simulink model "v7"  (R2023a)
settings: Solver=FixedStepAuto  StartTime=0.0  StopTime=Inf  RelTol=1e-3  EnableMultiTasking=on
undefined symbols (not defined in the file or in its folder): InputPWM, WheelSpeed
libraries: arduinolib x11, simulink x8, slpidlib x1, mobileRoboticsTrainingLib x1, arduinosensorlib x1
settings Model: ExtModeTrigDuration=2  Creator=friso  LastModifiedBy=friso
settings OptimizationCC: EnhancedBackFolding=on  PassReuseOutputArgsAs=Individual arguments  ZeroExternalMemoryAtStartup=off  ZeroInternalMemoryAtStartup=off  MaxStackSize=64  OptimizeBlockOrder=speed  DifferentSizesBufferReuse=on  OptimizationCustomize=off  EfficientTunableParamExpr=on
settings DebuggingCC: ParameterTunabilityLossMsg=error  UnderSpecifiedDimensionMsg=warning
settings HardwareCC: ProdBitPerPointer=32  ProdBitPerSizeT=32  ProdBitPerPtrDiffT=32  ProdLargestAtomicInteger=Long  ProdLargestAtomicFloat=Double  ProdWordSize=32  ProdHWDeviceType=ARM Compatible->ARM Cortex  UseEmbeddedCoderFeatures=off
settings SFSimCC: MATLABDynamicMemAlloc=off
settings RTWCC: Description=Embedded Coder  SystemTargetFile=ert.tlc  HardwareBoard=Arduino Nano 33 IoT  TemplateMakefile=ert_default_tmf  Toolchain=Arduino ARM  BuildConfiguration=Faster Runs
settings CodeAppCC: ForceParamTrailComments=on  IgnoreCustomStorageClasses=off  OperatorAnnotations=on  SimulinkDataObjDesc=on  SFDataObjDesc=on  InsertBlockDesc=on
settings ERTTargetCC: SupportContinuousTime=on  SupportNonInlinedSFcns=on  SupportVariableSizeSignals=on  ExtModeTransport=3  ExtModeStaticAlloc=on  ExtModeAutomaticAllocSize=off  ExtModeStaticAllocSize=8192  ExtModeMexFile=ext_xcp  ExtModeIntrfLevel=Level2 - Open

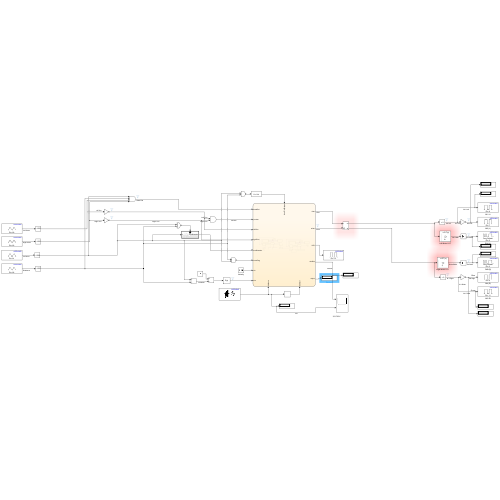
[thumbnail: Simulink's stored preview of the top-level diagram]
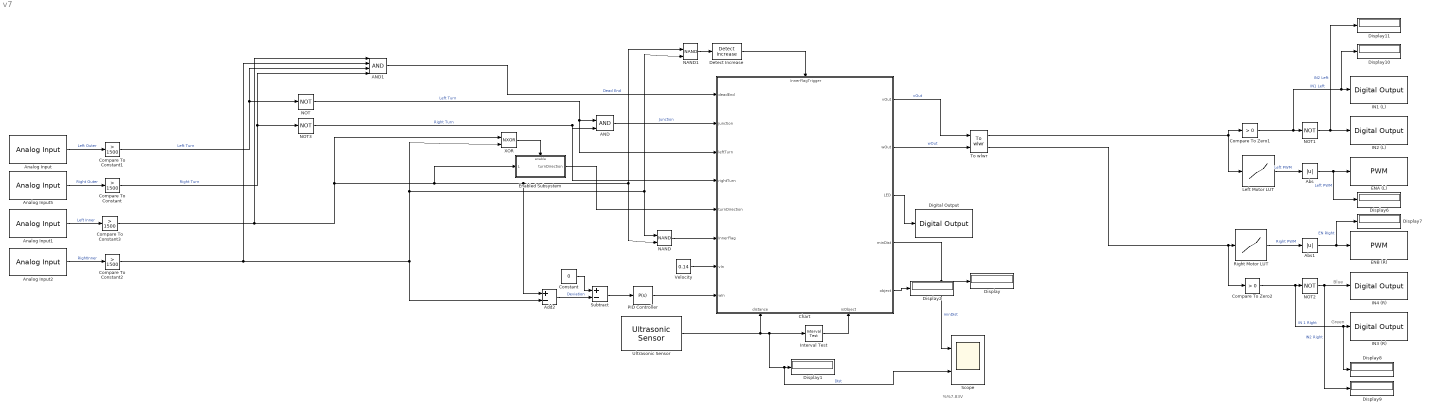
== system v7 ==
  note: %%7.83V
  note: Blue
  note: Green
  AND : Logic  IconShape=distinctive  AllPortsSameDT=off  OutDataTypeStr=boolean
  AND1 : Logic  Inputs=4  IconShape=distinctive  AllPortsSameDT=off  OutDataTypeStr=boolean
  Abs : Abs  SaturateOnIntegerOverflow=off
  Abs1 : Abs  SaturateOnIntegerOverflow=off
  Add2 : Sum  Inputs=+-  OutDataTypeStr=single
  Analog Input : arduinolib/Analog Input  pinNumber=0  ReadResultsOnly=off  ConversionTriggerSource=Software  ExternalTriggerType=uint32( 0 )  OutputDataType=uint16  EnableConversionCompleteNotify=off  EnableOuputStatus=off  SampleTime=-1  blockPlatform=arduino
  Analog Input1 : arduinolib/Analog Input  pinNumber=1  ReadResultsOnly=off  ConversionTriggerSource=Software  ExternalTriggerType=uint32( 0 )  OutputDataType=uint16  EnableConversionCompleteNotify=off  EnableOuputStatus=off  SampleTime=-1  blockPlatform=arduino
  Analog Input2 : arduinolib/Analog Input  pinNumber=2  ReadResultsOnly=off  ConversionTriggerSource=Software  ExternalTriggerType=uint32( 0 )  OutputDataType=uint16  EnableConversionCompleteNotify=off  EnableOuputStatus=off  SampleTime=-1  blockPlatform=arduino
  Analog Input5 : arduinolib/Analog Input  pinNumber=3  ReadResultsOnly=off  ConversionTriggerSource=Software  ExternalTriggerType=uint32( 0 )  OutputDataType=uint16  EnableConversionCompleteNotify=off  EnableOuputStatus=off  SampleTime=-1  blockPlatform=arduino
  Chart : Stateflow chart  TreatAsAtomicUnit=on
      settings: PortSchema="{\"entries\":[{\"content\":{\"sides\":[{\"content\":{\"connectorIds\":[\"In2\",\"In3\",\"In4\",\"In5\",\"In6\",\"In7\",\"In8\",\"In9\"]},\"type\":\"ConnectorPlacement.EquallySpacedRectSide\",\"uuid\":\"48d79888-744e-426e-80fd-4006989ca9f3\"},{\"content\":{\"connectorIds\":[\"Out2\",\"Out1\",\"Out3\",\"Out4\",\"Out5\"],\"side\":\"RIGHT\"},\"type\":\"ConnectorPlacement.EquallySpacedRectSide\",\"uuid\":\"a2b0e608-2864-4100-97ad-f114c331665e\"},{\"content\":{\"connectorIds\":[\"In1\"],\"side\":\"TOP\"},\"type\":\"ConnectorPlacement.EquallySpacedRectSide\",\"uuid\":\"9d579ed5-8468-4bce-b242-faef1fc44e90\"},{\"content\":{\"connectorIds\":[\"In11\",\"In10\"],\"side\":\"BOTTOM\"},\"type\":\"ConnectorPlacement.EquallySpacedRectSide\",\"uuid\":\"6fbdcd2a-7733-4dd1-bf5b-236cc3dcd5fd\"}]},\"type\":\"ConnectorPlacement.EquallySpacedConnector\",\"uuid\":\"bb2fff07-f9d5-40d5-a86f-bb5d79581747\"}],\"packageUris\":[\"http://schema.mathworks.com/mf0/Connector/R2020b\"],\"version\":\"1.0\"}"
  Compare To Constant{,1..3} (4 alike) : simulink/Logic and Bit Operations/Compare To Constant  relop=>  const=1500  OutDataTypeStr=uint8
  Compare To Zero1 : simulink/Logic and Bit Operations/Compare To Zero  relop=>  OutDataTypeStr=boolean
  Compare To Zero2 : simulink/Logic and Bit Operations/Compare To Zero  relop=>  OutDataTypeStr=boolean
  Constant : Constant  Value=0
  Detect Increase : simulink/Logic and Bit Operations/Detect Increase  vinit=0.0  OutDataTypeStr=boolean
  Digital Output : arduinolib/Digital Output  pinNumber=13  Direction=output  blockPlatform=arduino
  Display{,1..2,6..11} (9 alike) : Display
  ENA (L) : arduinolib/PWM  pinNumber=5  frequencyType=Default  desiredFrequency=490.2  achievableFrequency=490.2
  ENB (R) : arduinolib/PWM  pinNumber=3  frequencyType=Default  desiredFrequency=490.2  achievableFrequency=490.2
  Enabled Subsystem : Subsystem  TreatAsAtomicUnit=on
  IN1 (L) : arduinolib/Digital Output  pinNumber=9  Direction=output  blockPlatform=arduino
  IN2 (L) : arduinolib/Digital Output  pinNumber=7  Direction=output  blockPlatform=arduino
  IN3 (R) : arduinolib/Digital Output  pinNumber=11  Direction=output  blockPlatform=arduino
  IN4 (R) : arduinolib/Digital Output  pinNumber=6  Direction=output  blockPlatform=arduino
  Interval Test : simulink/Logic and Bit Operations/Interval Test  IntervalClosedRight=on  uplimit=0.5  IntervalClosedLeft=off  lowlimit=0  OutDataTypeStr=boolean
  Left Motor LUT : Lookup_n-D  NumberOfTableDimensions=1  BreakpointsForDimension1=WheelSpeed  Table=InputPWM  InterpMethod=Nearest  ExtrapMethod=Clip  InternalRulePriority=Speed  RndMeth=Simplest
  NAND : Logic  Operator=NAND  IconShape=distinctive  AllPortsSameDT=off  OutDataTypeStr=boolean
  NAND1 : Logic  Operator=NAND  IconShape=distinctive  AllPortsSameDT=off  OutDataTypeStr=boolean
  NOT{,1..3} (4 alike) : Logic  Operator=NOT  IconShape=distinctive  AllPortsSameDT=off  OutDataTypeStr=boolean
  PID Controller : slpidlib/PID Controller  Controller=P  Form=Parallel  TimeDomain=Continuous-time  UseExternalTs=off  SampleTime=-1  IntegratorMethod=Forward Euler  FilterMethod=Forward Euler  ControllerParametersSource=internal  P=0.87  I=1  UseKiTs=off  D=0  N=100  UseFilter=on  TunerSelectOption=Transfer Function Based (PID Tuner App)  InitialConditionSource=internal  InitialConditionForIntegrator=0  InitialConditionForFilter=0  DifferentiatorICPrevScaledInput=0  ExternalReset=none  TrackingMode=off  Kt=1  LimitOutput=off  SatLimitsSource=internal  UpperSaturationLimit=inf  LowerSaturationLimit=-inf  LinearizeAsGain=on  AntiWindupMode=none  Kb=1  LimitIntegrator=off  UpperIntegratorSaturationLimit=inf  LowerIntegratorSaturationLimit=-inf  POutMin=[]  POutMax=[]  IOutMin=[]  IOutMax=[]  DOutMin=[]  DOutMax=[]  NOutMin=[]  NOutMax=[]  SumOutMin=[]  SumOutMax=[]  SaturationOutMin=[]  SaturationOutMax=[]  PParamMin=[]  PParamMax=[]  IParamMin=[]  IParamMax=[]  DParamMin=[]  DParamMax=[]  NParamMin=[]  NParamMax=[]  KbParamMin=[]  KbParamMax=[]  KtParamMin=[]  KtParamMax=[]  KbOutMin=[]  KbOutMax=[]  KtOutMin=[]  KtOutMax=[]  IntegratorOutMin=[]  IntegratorOutMax=[]  FilterOutMin=[]  FilterOutMax=[]  SumI1OutMin=[]  SumI1OutMax=[]  SumI2OutMin=[]  SumI2OutMax=[]  SumI3OutMin=[]  SumI3OutMax=[]  SumI4OutMin=[]  SumI4OutMax=[]  SumDOutMin=[]  SumDOutMax=[]  DifferentiatorOutMin=[]  DifferentiatorOutMax=[]  FilterDiffOutCoefMin=[]  FilterDiffOutCoefMax=[]  ReciprocalOutMin=[]  ReciprocalOutMax=[]  SumDenOutMin=[]  SumDenOutMax=[]  SumNumOutMin=[]  SumNumOutMax=[]  DivideOutMin=[]  DivideOutMax=[]  UdiffTsProdOutMin=[]  UdiffTsProdOutMax=[]  NTsProdOutMin=[]  NTsProdOutMax=[]  UintegralTsProdOutMin=[]  UintegralTsProdOutMax=[]  UngainTsProdOutMin=[]  UngainTsProdOutMax=[]  ClampingZeroOutDataTypeStr=Inherit: Inherit via back propagation  ClampingZeroOutMin=[]  ClampingZeroOutMax=[]  FilterDenConstantOutDataTypeStr=Inherit: Inherit via back propagation  FilterDenConstantOutMin=[]  FilterDenConstantOutMax=[]  PCopyOutDataTypeStr=Inherit: Inherit via back propagation  PCopyOutMin=[]  PCopyOutMax=[]  NCopyOutDataTypeStr=Inherit: Inherit via back propagation  NCopyOutMin=[]  NCopyOutMax=[]  IntegratorContinuousStateAttributes=''  IntegratorStateMustResolveToSignalObject=off  IntegratorRTWStateStorageClass=Auto  FilterContinuousStateAttributes=''  FilterStateMustResolveToSignalObject=off  FilterRTWStateStorageClass=Auto  ParallelPVariant=InternalParameters  IdealPVariant=Disabled  IVariant=Disabled  DVariant=Disabled  IntegratorVariant=Disabled  SatVariant=Disabled  AWVariant=Disabled  PCopyVariant=Disabled  TRVariant=Disabled  FdbkBlocksVariant=Forward  IdealPFdbkVariant=Disabled  SatFdbkVariant=Disabled  DerivativeFilterVariant=Disabled  NVariant=Disabled  NCopyVariant=Disabled_SignalSpec  FilterICVariant=Disabled  IntegratorICVariant=Disabled  ExternalResetVariant=Disabled  TRSumVariant=Passthrough  SumFdbkVariant=Disabled  SumVariant=Passthrough_P  TsampFilterVariant=InternalTs  TsampNgainVariant=Passthrough  TsampIntegralVariant=Disabled_SignalSpec  ExternalSaturationOutDataTypeStr=Inherit: Same as second input
  Right Motor LUT : Lookup_n-D  NumberOfTableDimensions=1  BreakpointsForDimension1=WheelSpeed  Table=InputPWM  InterpMethod=Nearest  ExtrapMethod=Clip  InternalRulePriority=Speed  RndMeth=Simplest
  Scope : Scope  NumInputPorts=2
  Subtract : Sum  Inputs=+-
  To wlwr : mobileRoboticsTrainingLib/To wlwr  axleLength=axleLength  wheelR=wheelR
  Ultrasonic Sensor : arduinosensorlib/Ultrasonic Sensor  NumSignalPins=2  TrigPin=2  EchoPin=12  SignalPin=3  SampleTime_=0.1  blockPlatform=ARDUINO
  Velocity : Constant  Value=0.14
  XOR : Logic  Operator=NXOR  IconShape=distinctive  AllPortsSameDT=off  OutDataTypeStr=boolean
  wires:
  NOT2/1 -> IN4 (R)/1, Display9/1  "IN2 Right"
  NOT1/1 -> Display11/1, IN2 (L)/1  "IN2 Left"
  Compare To Zero2/1 -> Display8/1, IN3 (R)/1, NOT2/1  "IN 1 RIght"
  Left Motor LUT/1 -> Abs/1  "Left PWM"
  Abs1/1 -> Display7/1, ENB (R)/1  "EN RIght"
  Abs/1 -> Display6/1, ENA (L)/1  "Left PWM"
  Right Motor LUT/1 -> Abs1/1  "Right PWM"
  To wlwr/1 -> Left Motor LUT/1, Compare To Zero1/1
  Compare To Zero1/1 -> Display10/1, IN1 (L)/1, NOT1/1  "IN1 Left"
  Chart/1(wOut) -> To wlwr/2  "wOut"
  Chart/2(vOut) -> To wlwr/1  "vOut"
  Velocity/1 -> Chart/8(vIn)
  Constant/1 -> Subtract/1
  AND1/1 -> Chart/2(deadEnd)  "Dead End"
  Analog Input1/1 -> Compare To Constant3/1  "Left Inner"
  Compare To Constant1/1 -> AND1/3, NOT/1  "Left Turn"
  AND/1 -> Chart/3(junction)  "Junction"
  Compare To Constant2/1 -> AND1/2, Add2/2, XOR/2, NAND1/2, NAND/1
  PID Controller/1 -> Chart/9(wIn)
  Analog Input/1 -> Compare To Constant1/1  "Left Outer"
  Add2/1 -> Subtract/2  "Deviation"
  Compare To Constant/1 -> AND1/4, NOT3/1  "Right Turn"
  Analog Input5/1 -> Compare To Constant/1  "Right Outer"
  Subtract/1 -> PID Controller/1
  Analog Input2/1 -> Compare To Constant2/1  "RightInner"
  Compare To Constant3/1 -> Add2/1, NAND1/1, NAND/2, Enabled Subsystem/1(L), XOR/1, AND1/1
  NOT/1 -> Chart/4(leftTurn), AND/1  "Left Turn"
  NOT3/1 -> Chart/5(rightTurn), AND/2  "Right Turn"
  Ultrasonic Sensor/1 -> Chart/11(distance), Scope/2, Display1/1, Interval Test/1  "DIst"
  Interval Test/1 -> Chart/10(isObject)
  To wlwr/2 -> Compare To Zero2/1, Right Motor LUT/1
  XOR/1 -> Enabled Subsystem/Enable
  Enabled Subsystem/1(turnDirection) -> Chart/6(turnDirection)
  NAND/1 -> Chart/7(InnerFlag)
  Detect Increase/1 -> Chart/1(InnerFlagTrigger)
  NAND1/1 -> Detect Increase/1
  Chart/3(LED) -> Digital Output/1
  Chart/4(minDist) -> Scope/1, Display/1  "minDist"
  Chart/5(object) -> Display2/1

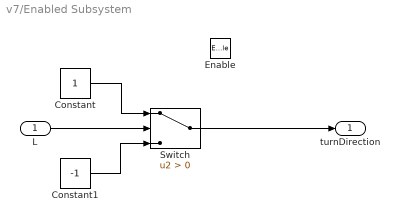
== system v7/Enabled Subsystem ==
  L : Inport
  Enable : EnablePort
  Constant : Constant
  Constant1 : Constant  Value=-1
  Switch : Switch  Criteria=u2 > Threshold  SaturateOnIntegerOverflow=off  InputSameDT=off
  turnDirection : Outport
  wires:
  Switch/1 -> turnDirection/1
  L/1 -> Switch/2
  Constant/1 -> Switch/1
  Constant1/1 -> Switch/3

== stateflow chart v7/Chart ==
  note: Slower: wIn: 0.72, vIn = 1.1
  state leftAfterJunction1
    entry:
    wOut = 1.5
    exit:
    prevTurn = -1
  state turnLeft1
    entry:
    vOut = 0.105 ;%% 0.105; % Small linear velocity
    wOut = wIn;
    during:
    on after(400, msec):
    vOut = 0;
    wOut = 1.5;% Counterclockwise
  state turnRight1
    entry:
    vOut = 0.105; % Small linear velocity Smaller: 0.105
    wOut = wIn;
    during:
    on after(400, msec):
    vOut = 0;
    wOut = -1.5;% Clockwise
  state leftAfterJunction
    % Seperate state due to
    % Timing difference
    entry:
    wOut = 1.5
    exit:;
    prevTurn = -1
  state turnLeft
    entry:
    vOut = 0.105 ; % Small linear velocity
    wOut = wIn;
    during:
    on after(400, msec):
    vOut = 0;
    wOut = 1.5; % Counterclockwise
  state turnRight
    entry:
    vOut = 0.105; % Small linear velocity
    wOut = wIn;
    during:
    on after(400, msec):
    vOut = 0;
    wOut = -1.5;% Clockwise
  state lineFollowing1
    entry, during:
    wOut = wIn  % from PI controller
    vOut = vIn % Constant
  state atJunction1
    % Various options
    entry:
    vOut, wOut = 0;
    during:
    vOut = vIn;
    exit:
    vOut = 0;
  state rightAfterJunction1
    entry:
    wOut = -1.5
    exit:
    prevTurn = 1;
  state returnToPath
    entry:
    vOut = 0; % No linear velocity
    wOut = 1.6
  state lineFollowing
    entry, during:
    wOut = wIn  % from PI controller
    vOut = vIn % Constant
  state atJunction
    % Various options
    entry:
    vOut, wOut = 0;
    during:
    vOut = vIn;
    exit:
    vOut = 0;
  state initialize
    entry:
    minDist = 100;
  state rightAfterJunction
    % Seperate state due to
    % Timing difference
    entry:
    wOut = -1.5
    exit:
    prevTurn = 1;
  state turnAround1
    entry:
    vOut = 0; % No linear velocity
    wOut = 1.6 % Slower: 1.35
    exit:
    LED = 0;
  state correction1
    entry:
    vOut = 0; % No linear velocity
    wOut = turnDirection*1.9 % Slower: 1.35
    % Turn direction dependent on which sensor was last on the line
  state finishLine
    entry:
    wOut = 0;
    vOut = 0
  state measureObject1
    % Record distance to object
    entry:
    LED = 1;
  state turnAround
    entry:
    vOut = 0; % No linear velocity
    wOut = 1.6 % Slower: 1.35
    exit:
    LED = 0;
  state correction
    entry:
    vOut = 0; % No linear velocity
    wOut = turnDirection*1.9 % Slower: 1.35
    % Turn direction dependent on which sensor was last on the line
  state measureObject
    % Record distance to object
    entry:
    LED = 1;
  state stop
    entry:
    vOut = 0;
    wOut = 0;
  (junction 332) -> (junction 331)
  (junction 330) -> (junction 332)
  (junction 331) -> leftAfterJunction1
  (junction 345) -> (junction 341)
  (junction 341) -> (junction 339)
  (junction 334) -> (junction 345)
  (junction 118) -> (junction 120)
  (junction 116) -> (junction 118)
  (junction 120) -> leftAfterJunction
  leftAfterJunction1 -> (junction 346)
  turnRight1 -> (junction 334) [order 1] : [leftTurn && before(400, msec)]
  turnLeft1 -> (junction 334) [order 1] : [rightTurn && before(400, msec)]
  turnRight1 -> (junction 346) [order 3]
  turnLeft1 -> (junction 346) [order 3]
  (junction 346) -> lineFollowing1 : [InnerFlagTrigger]
  (junction 79) -> (junction 83)
  (junction 83) -> (junction 84)
  (junction 76) -> (junction 79)
  turnLeft1 -> (junction 319) [order 2] : [InnerFlagTrigger && after(0.7, sec)]
      | {prevTurn = -1;}
  turnRight1 -> (junction 343) [order 2] : [InnerFlagTrigger && after(0.7, sec)]
      | {prevTurn = 1}
  (junction 319) -> lineFollowing1
  (junction 343) -> lineFollowing1
  leftAfterJunction -> (junction 64)
  (junction 320) -> turnRight1
  lineFollowing1 -> (junction 320) [order 4] : [rightTurn]
  (junction 322) -> turnLeft1 : [leftTurn]
  turnRight -> (junction 76) [order 1] : [leftTurn && before(400, msec)]
  turnLeft -> (junction 76) [order 1] : [rightTurn && before(400, msec)]
  turnRight -> (junction 64) [order 3]
  turnLeft -> (junction 64) [order 3]
  (junction 64) -> lineFollowing : [InnerFlagTrigger]
  lineFollowing1 -> atJunction1 [order 2] : [junction]
  lineFollowing1 -> (junction 322) [order 3]
  turnLeft -> (junction 297) [order 2] : [InnerFlagTrigger && after(0.6, sec)]
      | {prevTurn = -1}
  turnRight -> (junction 300) [order 2] : [InnerFlagTrigger && after(0.6, sec)]
      | {prevTurn = 1}
  (junction 297) -> lineFollowing
  (junction 300) -> lineFollowing
  (junction 339) -> atJunction1
  (junction 42) -> turnRight
  lineFollowing -> (junction 42) [order 4] : [rightTurn]
  (junction 72) -> turnLeft : [leftTurn]
  rightAfterJunction1 -> lineFollowing1 : [InnerFlagTrigger]
  atJunction1 -> rightAfterJunction1 [order 2] : [prevTurn ~= -1 && after(350, msec)]
  returnToPath -> lineFollowing1 : [InnerFlag && after(2.2, sec)]
  atJunction1 -> (junction 330) [order 3] : [prevTurn ~= 1 && after(350, msec)]
  (default) -> initialize
  turnAround1 -> lineFollowing1 : [InnerFlag && after(2, sec)]
  lineFollowing1 -> correction1 [order 1] : [deadEnd]
  correction1 -> lineFollowing1 : [InnerFlag]
  lineFollowing -> atJunction [order 2] : [junction]
  lineFollowing -> (junction 72) [order 3]
  initialize -> lineFollowing
  (junction 84) -> atJunction
  finishLine -> returnToPath
  atJunction1 -> measureObject1 [order 1] : [isObject]{object = distance}
  rightAfterJunction -> lineFollowing : [InnerFlagTrigger]
  atJunction -> rightAfterJunction [order 3] : [prevTurn ~= -1 && after(350, msec)]
  atJunction -> (junction 116) [order 4] : [prevTurn ~= 1 && after(350, msec)]
  turnAround -> lineFollowing : [InnerFlag && after(2, sec)]
  lineFollowing -> correction [order 1] : [deadEnd]
  correction -> lineFollowing : [InnerFlag]
  atJunction -> (junction 135) [order 2]
  atJunction -> measureObject [order 1] : [after(0.3, sec) && isObject]{object = distance}
  measureObject1 -> turnAround1 [order 2]
  (junction 135) -> finishLine : [junction && after(350, msec)]
  measureObject1 -> stop [order 1] : [object < 1.05*minDist]
  measureObject -> turnAround [order 2]
  measureObject -> (junction 377) [order 1] : [object < minDist && object > 0.025]{minDist = object}
  (junction 112) -> turnAround
  (junction 377) -> (junction 112)
  data: InnerFlagTrigger input; deadEnd input; junction input; leftTurn input; rightTurn input; turnDirection input; InnerFlag input; vIn input; wIn input; wOut output size=1; vOut output size=1; prevTurn local; isObject input; distance input [0.01..0.5]; LED output; minDist output; object output
